simulink model "VendingMachine"  (R2019b)
settings: Solver=VariableStepAuto  StartTime=0.0  StopTime=10.0  RelTol=1e-3
settings Model: Creator=ip  LastModifiedBy=ip

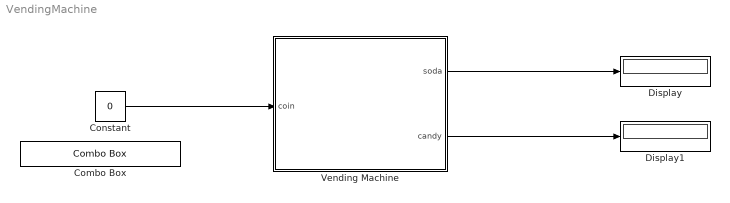
== system VendingMachine ==
  Combo Box : ComboBox  LabelPosition=Hide  SelectedLabel=No Coins
      settings: Values={{'No Coins', '1: Candy', '2: Soda'}, [0 1 2]}
  Constant : Constant  Value=0
  Display : Display
  Display1 : Display
  Vending Machine : Stateflow chart  BlockKeywords=__PRM__SERIALIZED__DATA__:Stateflow Chart,Stateflow Diagram  TreatAsAtomicUnit=on
  wires:
  Vending Machine/1(soda) -> Display/1
  Vending Machine/2(candy) -> Display1/1
  Constant/1 -> Vending Machine/1(coin)

== stateflow chart VendingMachine/Vending Machine ==
  state got_0
  state got_nickel
  state got_dime
  (default) -> got_0
  got_0 -> got_nickel [order 1] : [coin==1]{soda=0; candy=1;}
  got_nickel -> got_0 [order 2] : [coin==2]{soda=1;}
  got_dime -> got_0 [order 1] : [coin==1]{soda=1; candy=1;}
  got_0 -> got_dime [order 2] : [coin==2]{soda=0;}
  got_nickel -> got_dime [order 1] : [coin==1]{soda=0; candy=1;}
  got_dime -> got_nickel [order 2] : [coin==2]{soda=1;}
  data: soda output; candy output; coin input
